simulink model "Final_Project_Part_3_disturbances_Template"  (R2022a)
settings: Solver=VariableStepAuto  StartTime=0.0  StopTime=tspan  FixedStep=10  RelTol=1e-8
model workspace (MATLAB code in the model file):
  | mu = 398601; % km
  | Re = 6378.137; %km
values from neighbouring files (symbols this model uses):
  J = [812.04 0 0; 0 545.37 0; 0 0 627.71]    [A421_FinalProject_Pt5.m]    (also in A421_FinalProject_Pt6.m; Final_Project_Part_3_disturbances_torques.m; Final_Project_Pt4.m; hw5.m = diag([1200, 2000, 2800]))
  JD_0 = 2460390    [A421_FinalProject_Pt5.m]    (also in A421_FinalProject_Pt6.m; Final_Project_Part_3_disturbances.m; Final_Project_Part_3_disturbances_init_Template-1.m; Final_Project_Part_3_disturbances_init_Template.m)
  m_b = [0;0;-0.5]    [A421_FinalProject_Pt5.m]    (also in A421_FinalProject_Pt6.m; Final_Project_Pt4.m)
  r_ECI_0 = rECI    [A421_FinalProject_Pt5.m]    (also in A421_FinalProject_Pt6.m; Final_Project_Pt4.m)
  sun_ECI = [1;0;0]    [A421_FinalProject_Pt5.m]    (also in A421_FinalProject_Pt6.m; Final_Project_Part_3_disturbances_torques.m; Final_Project_Pt4.m)
  surfaceProperties = [Areas_1 cps_1 normals_1; Areas_2 cps_2 normals_2; Areas_3 cps_3 normals_3; Areas_4 cps_4 normals_4]    [A421_FinalProject_Pt5.m]    (also in A421_FinalProject_Pt6.m; Final_Project_Part_3_disturbances.m = [Areas cps normals]; Final_Project_Part_3_disturbances_init_Template-1.m = [Areas cps normals]; Final_Project_Part_3_disturbances_init_Template.m = [Areas cps normals])
  T_c = [0; 0; 0]    [A421_FinalProject_Pt5.m]    (also in A421_FinalProject_Pt6.m; Final_Project_Part_3_disturbances.m; Final_Project_Part_3_disturbances_init_Template-1.m; Final_Project_Part_3_disturbances_init_Template.m)
  v_ECI_0 = vECI    [A421_FinalProject_Pt5.m]    (also in A421_FinalProject_Pt6.m; Final_Project_Pt4.m)
settings Model: Creator=emehiel  LastModifiedBy=emehiel
settings SolverCC: AlgebraicLoopSolver=TrustRegion
settings DebuggingCC: UnconnectedInputMsg=warning  UnconnectedOutputMsg=warning  UnconnectedLineMsg=warning  SFMachineParentedDataDiag=warning

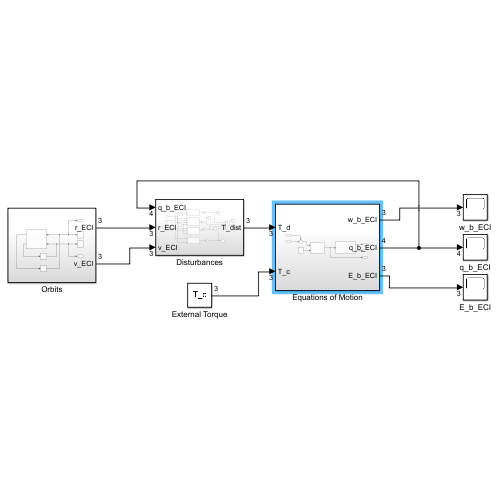
[thumbnail: Simulink's stored preview of the top-level diagram]
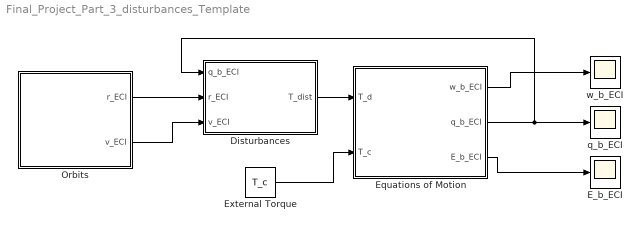
== system Final_Project_Part_3_disturbances_Template ==
  Disturbances : Subsystem
  E_b_ECI : Scope
  Equations of Motion : Subsystem
  External Torque : Constant  Value=T_c
  Orbits : Subsystem
  q_b_ECI : Scope
  w_b_ECI : Scope
  wires:
  Orbits/1(r_ECI) -> Disturbances/2(r_ECI)
  Orbits/2(v_ECI) -> Disturbances/3(v_ECI)
  Equations of Motion/2(q_b_ECI) -> Disturbances/1(q_b_ECI), q_b_ECI/1
  Equations of Motion/1(w_b_ECI) -> w_b_ECI/1
  Disturbances/1(T_dist) -> Equations of Motion/1(T_d)
  Equations of Motion/3(E_b_ECI) -> E_b_ECI/1
  External Torque/1 -> Equations of Motion/2(T_c)

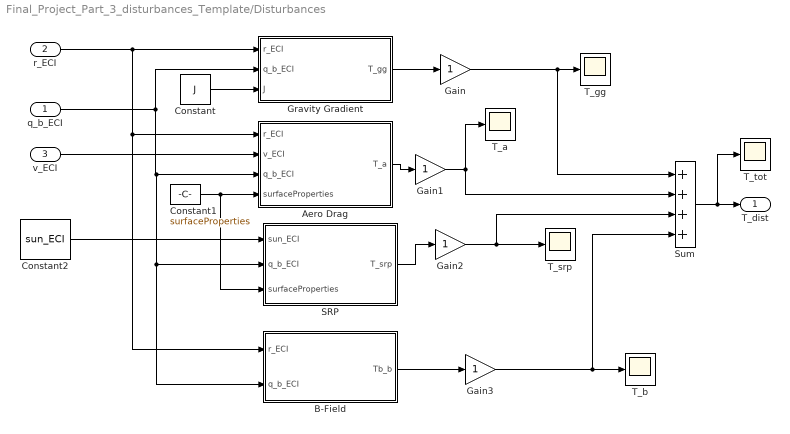
== system Final_Project_Part_3_disturbances_Template/Disturbances ==
  q_b_ECI : Inport
  r_ECI : Inport  Port=2
  v_ECI : Inport  Port=3
  Aero Drag : MATLAB Function  TreatAsAtomicUnit=on
  B-Field : Subsystem
  Constant : Constant  Value=J
  Constant1 : Constant  Value=surfaceProperties
  Constant2 : Constant  Value=sun_ECI
  Gain{,1..3} (4 alike) : Gain
  Gravity Gradient : MATLAB Function  TreatAsAtomicUnit=on
  SRP : MATLAB Function  TreatAsAtomicUnit=on
  Sum : Sum  Inputs=++++
  T_a : Scope
  T_b : Scope
  T_gg : Scope
  T_srp : Scope
  T_tot : Scope
  T_dist : Outport
  wires:
  Sum/1 -> T_tot/1, T_dist/1
  Aero Drag/1(T_a) -> Gain1/1
  Gravity Gradient/1(T_gg) -> Gain/1
  SRP/1(T_srp) -> Gain2/1
  Constant1/1 -> SRP/3(surfaceProperties), Aero Drag/4(surfaceProperties)
  v_ECI/1 -> Aero Drag/2(v_ECI)
  q_b_ECI/1 -> B-Field/2(q_b_ECI), SRP/2(q_b_ECI), Aero Drag/3(q_b_ECI), Gravity Gradient/2(q_b_ECI)
  Constant/1 -> Gravity Gradient/3(J)
  Constant2/1 -> SRP/1(sun_ECI)
  r_ECI/1 -> B-Field/1(r_ECI), Aero Drag/1(r_ECI), Gravity Gradient/1(r_ECI)
  B-Field/1(Tb_b) -> Gain3/1
  Gain/1 -> Sum/1, T_gg/1
  Gain1/1 -> Sum/2, T_a/1
  Gain2/1 -> Sum/3, T_srp/1
  Gain3/1 -> T_b/1, Sum/4

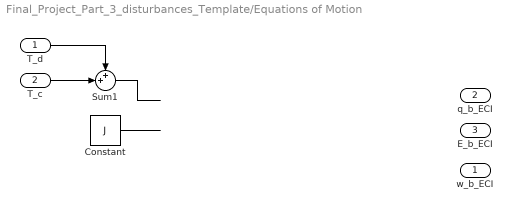
== system Final_Project_Part_3_disturbances_Template/Equations of Motion ==
  T_d : Inport
  T_c : Inport  Port=2
  Constant : Constant  Value=J
  Sum1 : Sum  Inputs=++|
  w_b_ECI : Outport  VectorParamsAs1DForOutWhenUnconnected=off
  q_b_ECI : Outport  Port=2  VectorParamsAs1DForOutWhenUnconnected=off
  E_b_ECI : Outport  Port=3  VectorParamsAs1DForOutWhenUnconnected=off
  wires:
  ? -> E_b_ECI/1
  Sum1/1 -> ?
  Constant/1 -> ?
  T_d/1 -> Sum1/1
  T_c/1 -> Sum1/2
  ? -> q_b_ECI/1
  ? -> w_b_ECI/1

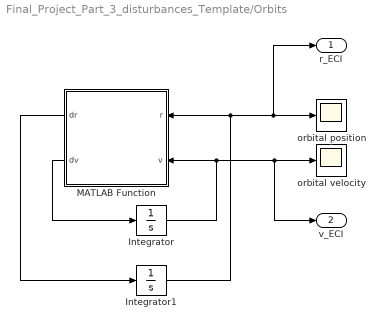
== system Final_Project_Part_3_disturbances_Template/Orbits ==
  Integrator : Integrator  InitialCondition=v_ECI_0
  Integrator1 : Integrator  InitialCondition=r_ECI_0
  MATLAB Function : MATLAB Function  TreatAsAtomicUnit=on
  orbital position : Scope
  orbital velocity : Scope
  r_ECI : Outport  VectorParamsAs1DForOutWhenUnconnected=off
  v_ECI : Outport  Port=2  VectorParamsAs1DForOutWhenUnconnected=off
  wires:
  Integrator/1 -> v_ECI/1, orbital velocity/1, MATLAB Function/2(v)
  Integrator1/1 -> r_ECI/1, orbital position/1, MATLAB Function/1(r)
  MATLAB Function/1(dr) -> Integrator1/1
  MATLAB Function/2(dv) -> Integrator/1

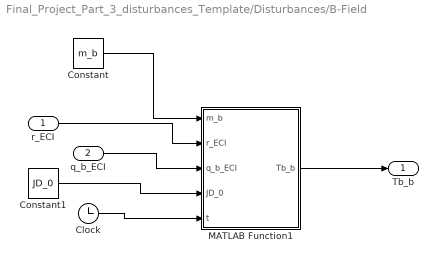
== system Final_Project_Part_3_disturbances_Template/Disturbances/B-Field ==
  r_ECI : Inport
  q_b_ECI : Inport  Port=2
  Clock : Clock
  Constant : Constant  Value=m_b  VectorParams1D=off
  Constant1 : Constant  Value=JD_0
  MATLAB Function1 : MATLAB Function  TreatAsAtomicUnit=on
  Tb_b : Outport
  wires:
  MATLAB Function1/1(Tb_b) -> Tb_b/1
  q_b_ECI/1 -> MATLAB Function1/3(q_b_ECI)
  r_ECI/1 -> MATLAB Function1/2(r_ECI)
  Clock/1 -> MATLAB Function1/5(t)
  Constant1/1 -> MATLAB Function1/4(JD_0)
  Constant/1 -> MATLAB Function1/1(m_b)

== matlab function Final_Project_Part_3_disturbances_Template/Disturbances/Gravity Gradient ==
  data: r_ECI input; T_gg output; q_b_ECI input; J input
function T_gg = gg_torque(r_ECI, q_b_ECI, J)

== matlab function Final_Project_Part_3_disturbances_Template/Disturbances/Aero Drag ==
  data: r_ECI input; v_ECI input; T_a output; q_b_ECI input; surfaceProperties input
function T_a = aero_drag_torque(r_ECI, v_ECI, q_b_ECI, surfaceProperties) 

% Convert v_ECI to v_b

% Calculate density using standard exponetial decay model (or model of your
% choice)

% Loop through all the surfaces of the MehielSat
for i = 1:length(surfaceProperties)
    % Find wetted area

    if A_wet > 0
        % Add to total torque from atmospheric drag
    end
end

== matlab function Final_Project_Part_3_disturbances_Template/Disturbances/SRP ==
  data: sun_ECI input; T_srp output; q_b_ECI input; surfaceProperties input
function T_srp  = SPR_torque(sun_ECI, q_b_ECI, surfaceProperties)

p_sun = 4.5e-6; %N/m (given)

== matlab function Final_Project_Part_3_disturbances_Template/Orbits/MATLAB Function ==
  data: r input; dr output; v input; dv output
function [dr,dv] = orbitalDynamics(r, v)
%#codegen

== matlab function Final_Project_Part_3_disturbances_Template/Disturbances/B-Field/MATLAB Function1 ==
  data: m_b input; r_ECI input; q_b_ECI input; Tb_b output; JD_0 input; t input
function Tb_b = WMM(m_b, r_ECI, q_b_ECI, JD_0, t)

% DGRF 2020 (given)
a = 6371.2; %km
g_11 = -1450.9; %nT
h_11 = 4652.5; %nT
g_10 = -29404.8; %nT
m_ECEF = a^3*[g_11; h_11; g_10];
